simulink model "TrayectoriaStateFlow"  (R2023b)
settings: Solver=FixedStepAuto  StartTime=0.0  StopTime=50  RelTol=1e-3  EnableMultiTasking=on
model workspace (MAT data in the model file):
  d = 0.223
settings Model: ExtModeTrigDuration=2  Creator=Manuel  LastModifiedBy=Manuel
settings OptimizationCC: EnhancedBackFolding=on  PassReuseOutputArgsAs=Individual arguments  ZeroExternalMemoryAtStartup=off  ZeroInternalMemoryAtStartup=off  MaxStackSize=64  OptimizeBlockOrder=speed  DifferentSizesBufferReuse=on  EfficientTunableParamExpr=on
settings DebuggingCC: ParameterTunabilityLossMsg=error
settings HardwareCC: ProdBitPerInt=16  ProdBitPerPointer=16  ProdBitPerSizeT=16  ProdBitPerPtrDiffT=16  ProdLargestAtomicFloat=None  ProdWordSize=8  ProdHWDeviceType=Atmel->AVR
settings SFSimCC: MATLABDynamicMemAlloc=off
settings RTWCC: Description=Embedded Coder  SystemTargetFile=ert.tlc  HardwareBoard=Arduino Mega 2560  TemplateMakefile=ert_default_tmf  Toolchain=Arduino AVR  BuildConfiguration=Faster Runs
settings CodeAppCC: ForceParamTrailComments=on  IgnoreCustomStorageClasses=off  OperatorAnnotations=on  SimulinkDataObjDesc=on  SFDataObjDesc=on  InsertBlockDesc=on
settings ERTTargetCC: SupportContinuousTime=on  SupportVariableSizeSignals=on  ExtModeTransport=3  ExtModeStaticAlloc=on  ExtModeAutomaticAllocSize=off  ExtModeStaticAllocSize=2048  ExtModeMexFile=ext_xcp  ExtModeIntrfLevel=Level2 - Open

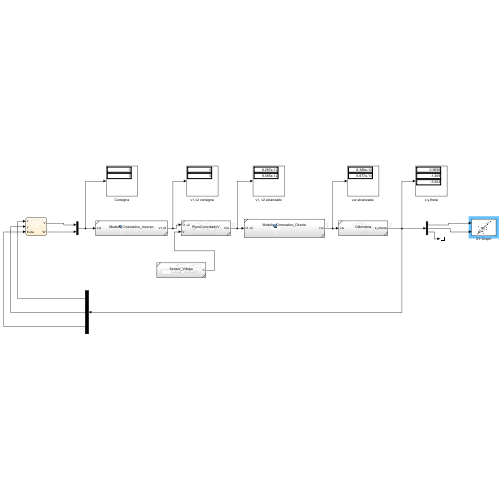
[thumbnail: Simulink's stored preview of the top-level diagram]
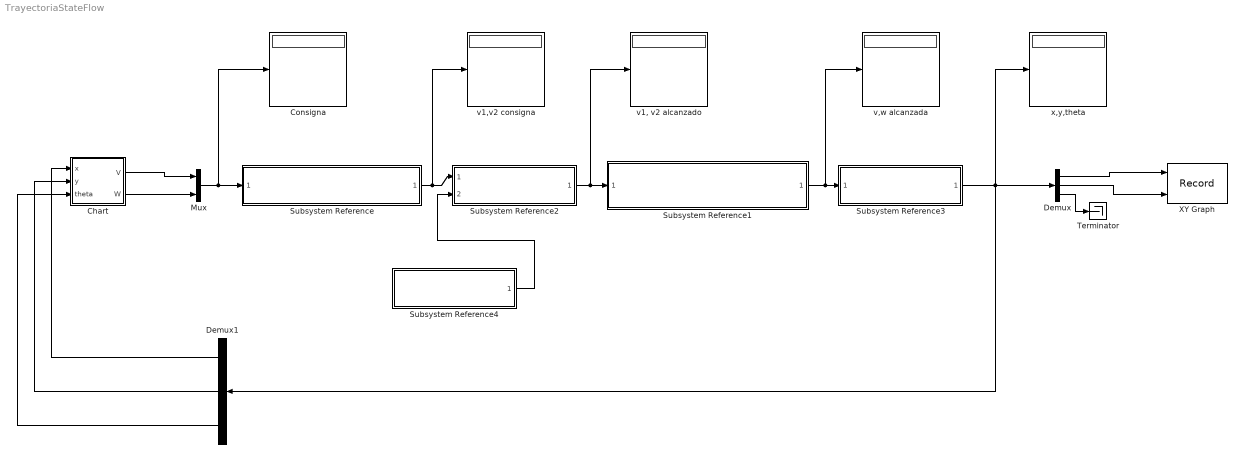
== system TrayectoriaStateFlow ==
  Chart : Stateflow chart  TreatAsAtomicUnit=on
  Consigna : Display
  Demux : Demux  Outputs=3
  Demux1 : Demux  Outputs=3
  Mux : Mux  Inputs=2
  Subsystem Reference : Subsystem  ReferencedSubsystem=Modelo_Cinematico_Inverso
  Subsystem Reference1 : Subsystem  ReferencedSubsystem=Modelo_Cinematico_Directo
  Subsystem Reference2 : Subsystem  ReferencedSubsystem=PieroControladoV
  Subsystem Reference3 : Subsystem  ReferencedSubsystem=Odometria
  Subsystem Reference4 : Subsystem  ReferencedSubsystem=Sensor_Voltaje
  Terminator : Terminator
  XY Graph : Record  FileSettingsInternal="{\"entries\":[{\"content\":{\"excelSettings\":{\"content\":{},\"type\":\"Streamout.ExcelSettings\"}},\"type\":\"Streamout.FileSettingStorage\",\"uuid\":\"\"}],\"packageUris\":[\"http:\\/\\/schema.mathworks.com\\/mf0\\/streamout_blocks\\/R2020a\"],\"version\":\"1.0\"}"  Layout=[1 1]  SignalsInternal="{\"entries\":[{\"content\":{\"signals\":[{\"content\":{\"blockPath\":[],\"dimensions\":[1],\"domain\":\"\",\"lineColor\":\"#a2142f\",\"plots\":[1],\"port\":1,\"sid\":[\"\"],\"signalID\":311694,\"signalName\":\"Demux:1\"},\"type\":\"RecordBlkView.Signal\",\"uuid\":\"\"},{\"content\":{\"blockPath\":[],\"dimensions\":[1],\"domain\":\"\",\"lineColor\":\"#139fff\",\"plots\":[1],\"port\":2,\"sid\":[\"\"],\"signalID\":311698,\"signalName\":\"Demux:2\"},\"type\":\"RecordBlkView.Signal\",\"uuid\":\"\"}]},\"type\":\"RecordBlkView.InputSignals\",\"uuid\":\"\"}],\"packageUris\":[\"http:\\/\\/schema.mathworks.com\\/mf0\\/streamout_blocks\\/R2020a\"],\"version\":\"1.0\"}"  VisualizationBindings="{\"xyplotplugin\":{\"info\":[{\"series\":[{\"bindingParametersList\":[{\"parameter\":\"X-Axis\",\"signalID\":311694,\"signalName\":\"Demux:1\"},{\"parameter\":\"Y-Axis\",\"signalID\":311698,\"signalName\":\"Demux:2\"}],\"seriesID\":39789}],\"subplotID\":1}]}}"  CompatibilityTag=XY
  "v,w alcanzada " : Display
  "v1, v2 alcanzado" : Display
  v1,v2 consigna : Display
  x,y,theta : Display
  wires:
  Subsystem Reference1/1 -> "v,w alcanzada "/1, Subsystem Reference3/1
  Subsystem Reference/1 -> v1,v2 consigna/1, Subsystem Reference2/1
  Subsystem Reference2/1 -> "v1, v2 alcanzado"/1, Subsystem Reference1/1
  Subsystem Reference3/1 -> Demux1/1, Demux/1, x,y,theta/1
  Demux/1 -> XY Graph/1
  Demux/2 -> XY Graph/2
  Demux/3 -> Terminator/1
  Mux/1 -> Consigna/1, Subsystem Reference/1
  Chart/1(V) -> Mux/1
  Chart/2(W) -> Mux/2
  Demux1/1 -> Chart/1(x)
  Demux1/2 -> Chart/2(y)
  Demux1/3 -> Chart/3(theta)
  Subsystem Reference4/1 -> Subsystem Reference2/2

== stateflow chart TrayectoriaStateFlow/Chart ==
  state GiroIzquierda2
    entry:
    V=0.08;
    W=-pi/6
  state Marcha2
    entry:
    V=0.3;
    W=0;
  state GiroIzquierda1
    entry:
    V=0.08;
    W=-pi/6;
  state Marcha3
    entry:
    V=0.3;
    W=0;
  state Marcha1
    entry:
    V=0.3;
    W=0;
  state Fin
    entry:
    V=0;
    W=0;
  state Inicio
    entry:
    V=0;
    W=0;
  Marcha2 -> GiroIzquierda2 : [y<-1.2]
  GiroIzquierda1 -> Marcha2 : [theta<-pi/2]
  GiroIzquierda2 -> Marcha3 : [theta<-pi]
  Marcha1 -> GiroIzquierda1 : [x>2.1]
  Marcha3 -> Fin : [x<1]
  Inicio -> Marcha1 : after(1,sec)
  (default) -> Inicio
  data: V output double size=1; W output double size=1; x input double size=1; y input double size=1; theta input double size=1
